simulink model "sfcndemo_varsize"  (Simulink 7.6)
settings: Solver=FixedStepDiscrete  StartTime=0.0  StopTime=2.0  RelTol=1e-3
libraries: simulink x1
settings Model: Creator=The MathWorks Inc.
settings DataIOCC: SaveFormat=StructureWithTime
settings SFSimCC: SimParseCustomCode=off

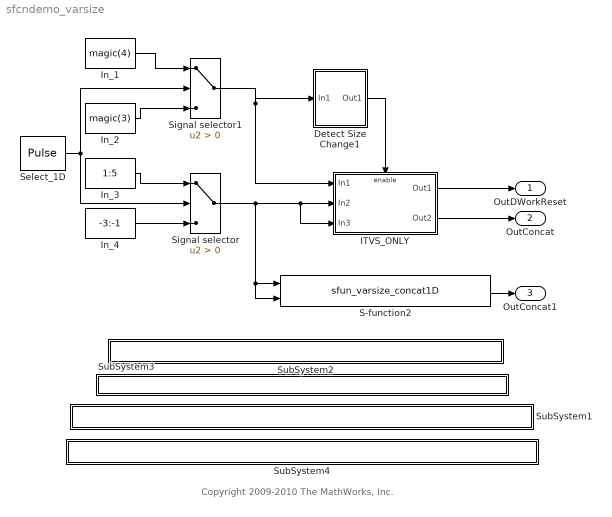
== system sfcndemo_varsize ==
  note: Copyright 2009-2010 The MathWorks, Inc.
  Detect Size Change1 : Subsystem
  ITVS_ONLY : Subsystem  TreatAsAtomicUnit=on
  In_1 : Constant  Value=magic(4)
  In_2 : Constant  Value=magic(3)
  In_3 : Constant  Value=1:5
  In_4 : Constant  Value=-3:-1
  S-function2 : S-Function  FunctionName=sfun_varsize_concat1D  EnableBusSupport=off
  Select_1D : DiscretePulseGenerator  Period=8  PulseWidth=4  SampleTime=.2
  Signal selector : Switch  Criteria=u2 > Threshold  AllowDiffInputSizes=on
  Signal selector1 : Switch  Criteria=u2 > Threshold  AllowDiffInputSizes=on
  SubSystem1 : Subsystem  mask{filename=sfun_varsize_holdStatesUntilReset.c}
      mask init:
      | x=sfundemo_maskdisp;
      settings: AttributesFormatString=\n  OpenFcn=sfundemo_openfcn
      mask Display: disp(x);
  SubSystem2 : Subsystem  mask{filename=sfun_varsize_concat1D.c}
      mask init:
      | x=sfundemo_maskdisp;
      settings: AttributesFormatString=\n  OpenFcn=sfundemo_openfcn
      mask Display: disp(x);
  SubSystem3 : Subsystem  mask{filename=sfun_varsize_concat1D.tlc}
      mask init:
      | x=sfundemo_maskdisp;
      settings: AttributesFormatString=\n  OpenFcn=sfundemo_openfcn
      mask Display: disp(x);
  SubSystem4 : Subsystem  mask{filename=sfun_varsize_holdStatesUntilReset.tlc}
      mask init:
      | x=sfundemo_maskdisp;
      settings: AttributesFormatString=\n  OpenFcn=sfundemo_openfcn
      mask Display: disp(x);
  OutDWorkReset : Outport
  OutConcat : Outport  Port=2
  OutConcat1 : Outport  Port=3
  wires:
  ITVS_ONLY/1(Out1) -> OutDWorkReset/1
  In_3/1 -> Signal selector/1
  Select_1D/1 -> Signal selector/2, Signal selector1/2
  In_4/1 -> Signal selector/3
  Signal selector/1 -> S-function2/1, S-function2/2, ITVS_ONLY/2(In2), ITVS_ONLY/3(In3)
  ITVS_ONLY/2(Out2) -> OutConcat/1
  S-function2/1 -> OutConcat1/1
  In_2/1 -> Signal selector1/3
  Signal selector1/1 -> ITVS_ONLY/1(In1), Detect Size Change1/1(In1)
  Detect Size Change1/1(Out1) -> ITVS_ONLY/Enable
  In_1/1 -> Signal selector1/1

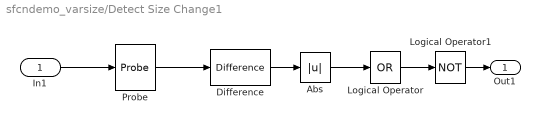
== system sfcndemo_varsize/Detect Size Change1 ==
  In1 : Inport
  Abs : Abs
  Difference : simulink/Discrete/Difference  SystemSampleTime=-1  ICPrevInput=[4 4]  OutMin=[]  OutMax=[]  OutDataType=fixdt(1, 16)  OutScaling=2^-10  DoSatur=off
  Logical Operator : Logic  Operator=OR  Inputs=1  AllPortsSameDT=off  OutDataTypeStr=boolean
  Logical Operator1 : Logic  Operator=NOT  Inputs=1  AllPortsSameDT=off  OutDataTypeStr=boolean
  Probe : Probe  ProbeWidth=off  ProbeSampleTime=off  ProbeComplexSignal=off  ProbeSignalDimensions=on
  Out1 : Outport
  wires:
  Logical Operator/1 -> Logical Operator1/1
  Abs/1 -> Logical Operator/1
  In1/1 -> Probe/1
  Probe/1 -> Difference/1
  Difference/1 -> Abs/1
  Logical Operator1/1 -> Out1/1

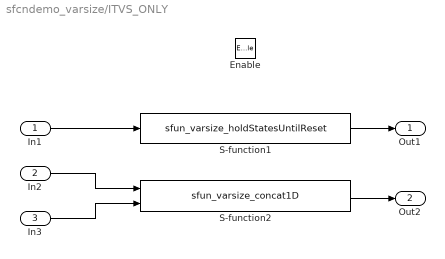
== system sfcndemo_varsize/ITVS_ONLY ==
  In1 : Inport
  In2 : Inport  Port=2
  In3 : Inport  Port=3
  Enable : EnablePort  StatesWhenEnabling=reset
  S-function1 : S-Function  FunctionName=sfun_varsize_holdStatesUntilReset  EnableBusSupport=off
  S-function2 : S-Function  FunctionName=sfun_varsize_concat1D  EnableBusSupport=off
  Out1 : Outport
  Out2 : Outport  Port=2
  wires:
  S-function1/1 -> Out1/1
  In1/1 -> S-function1/1
  In2/1 -> S-function2/1
  In3/1 -> S-function2/2
  S-function2/1 -> Out2/1

== system sfcndemo_varsize/SubSystem1 ==

== system sfcndemo_varsize/SubSystem2 ==

== system sfcndemo_varsize/SubSystem3 ==

== system sfcndemo_varsize/SubSystem4 ==
